simulink model "sampleModel1810_2"  (R2023a)
settings: Solver=VariableStepAuto  StartTime=0.0  StopTime=10.0  RelTol=1e-3
libraries: hdlsllib x6, simulink x4
settings Model: Creator=user1  LastModifiedBy=user1

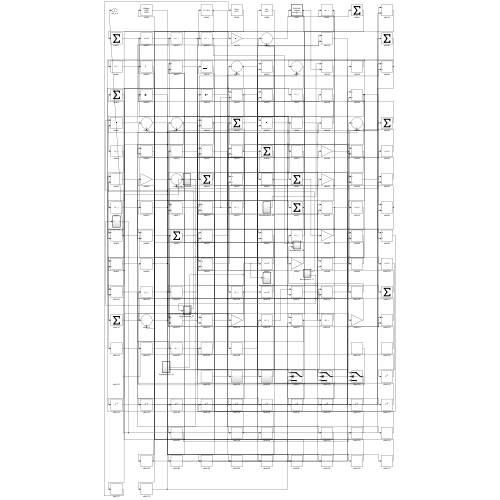
[thumbnail: Simulink's stored preview of the top-level diagram]
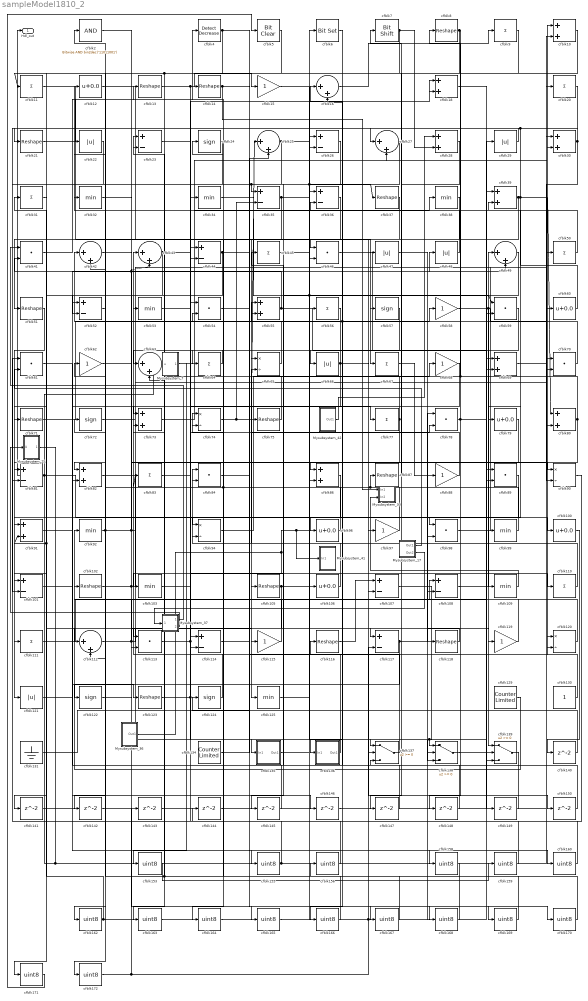
== system sampleModel1810_2 ==
  Mysubsystem_17 : Subsystem  TreatAsAtomicUnit=on  RTWFcnName=Mysubsystem_17
      settings: RTWFcnNameOpts=User specified  RTWFileNameOpts=Use function name
  Mysubsystem_25 : Subsystem  TreatAsAtomicUnit=on  RTWFcnName=Mysubsystem_25
      settings: RTWFcnNameOpts=User specified  RTWFileNameOpts=Use function name
  Mysubsystem_30 : Subsystem  TreatAsAtomicUnit=on  RTWFcnName=Mysubsystem_30
      settings: RTWFcnNameOpts=User specified  RTWFileNameOpts=Use function name
  Mysubsystem_36 : Subsystem  TreatAsAtomicUnit=on  RTWFcnName=Mysubsystem_36
      settings: RTWFcnNameOpts=User specified  RTWFileNameOpts=Use function name
  Mysubsystem_37 : Subsystem  TreatAsAtomicUnit=on  RTWFcnName=Mysubsystem_37
      settings: RTWFcnNameOpts=User specified  RTWFileNameOpts=Use function name
  Mysubsystem_41 : Subsystem  TreatAsAtomicUnit=on  RTWFcnName=Mysubsystem_41
      settings: RTWFcnNameOpts=User specified  RTWFileNameOpts=Use function name
  Mysubsystem_42 : Subsystem  TreatAsAtomicUnit=on  RTWFcnName=Mysubsystem_42
      settings: RTWFcnNameOpts=User specified  RTWFileNameOpts=Use function name
  Mysubsystem_7 : Subsystem  TreatAsAtomicUnit=on  RTWFcnName=Mysubsystem_7
      settings: RTWFcnNameOpts=User specified  RTWFileNameOpts=Use function name
  cfblk{10,18,28,30,39,55,69,73,80,82,86,91} (12 alike) : Sum  OutDataTypeStr=uint8
  cfblk{12,60,79,96,100,106} (6 alike) : Bias  Bias=0.0  SaturateOnIntegerOverflow=off
  cfblk{23,26,35..36,44,52,81,101,107..108,114,117} (12 alike) : Sum  Inputs=+-  OutDataTypeStr=uint8
  cfblk{8,13..14,21,37,51,71,75,87,102,105,116,118,123} (14 alike) : Reshape
  cfblk{32,34,38,53,92,99,103,109,125} (9 alike) : MinMax  OutDataTypeStr=uint8
  cfblk{9,11,20,31,45,50,56,64,67,77,83,110..111} (13 alike) : Sum  Inputs=+  OutDataTypeStr=uint8
  cfblk{16,25,27,42..43,49,63,112} (8 alike) : Sum  Inputs=|++  OutDataTypeStr=uint8
  cfblk{41,46,54,59,61,70,78,84,89,98,113} (11 alike) : DotProduct  OutDataTypeStr=uint8
  cfblk{15,58,62,68,88,97,115,119} (8 alike) : Gain  OutDataTypeStr=uint8
  cfblk{65,74,90,94,120} (5 alike) : Product  Inputs=*/  OutDataTypeStr=uint8  RndMeth=Zero  SaturateOnIntegerOverflow=on
  cfblk{22,29,47..48,66,121} (6 alike) : Abs  OutDataTypeStr=uint8  SaturateOnIntegerOverflow=off
  cfblk{24,57,72,122,124} (5 alike) : Signum
  cfblk129 : hdlsllib/Sources/Counter Limited  uplimit=7  tsamp=-1
  cfblk130 : Constant  OutDataTypeStr=uint8  SampleTime=-1
  cfblk131 : Ground
  cfblk134 : hdlsllib/Sources/Counter Limited  uplimit=7  tsamp=-1
  cfblk135 : Subsystem
      settings: LibrarySourceBlock=|
      | hdlsllib/Ports &
      | Subsystems/Subsystem
  cfblk136 : Subsystem
      settings: LibrarySourceBlock=|
      | hdlsllib/Ports &
      | Subsystems/Subsystem
  cfblk137 : Switch  OutDataTypeStr=uint8  SaturateOnIntegerOverflow=off  InputSameDT=off
  cfblk138 : Switch  OutDataTypeStr=uint8  SaturateOnIntegerOverflow=off  InputSameDT=off
  cfblk139 : Switch  OutDataTypeStr=uint8  SaturateOnIntegerOverflow=off  InputSameDT=off
  cfblk{140..150} (11 alike) : Delay  SampleTime=1
  cfblk{153,155..156,158..160,162..172} (17 alike) : DataTypeConversion  OutDataTypeStr=uint8  SaturateOnIntegerOverflow=off  RndMeth=Floor
  cfblk2 : simulink/Logic and Bit Operations/Bitwise Operator  logicop=AND  UseBitMask=on  BitMask=bin2dec('11011001')  BitMaskRealWorld=Stored Integer
      settings: LibrarySourceBlock=|
      | hdlsllib/Logic and Bit
      | Operations/Bitwise
      | Operator
  cfblk4 : simulink/Logic and Bit Operations/Detect Decrease  vinit=0.0  OutDataTypeStr=uint8
      settings: LibrarySourceBlock=|
      | hdlsllib/Logic and Bit
      | Operations/Detect
      | Decrease
  cfblk5 : simulink/Logic and Bit Operations/Bit Clear  iBit=0
      settings: LibrarySourceBlock=|
      | hdlsllib/Logic and Bit
      | Operations/Bit Clear
  cfblk6 : simulink/Logic and Bit Operations/Bit Set  iBit=0
      settings: LibrarySourceBlock=|
      | hdlsllib/Logic and Bit
      | Operations/Bit Set
  cfblk7 : hdlsllib/Logic and Bit Operations/Bit Shift  mode=Shift Left Logical  N=0
  Hdl_out : Outport  OutDataTypeStr=uint8
  wires:
  cfblk116/1 -> cfblk107/1
  cfblk82/1 -> cfblk135/1(In1)
  cfblk9/1 -> cfblk11/1, cfblk73/1
  cfblk65/1 -> cfblk42/1
  cfblk130/1 -> cfblk10/1
  cfblk67/1 -> cfblk88/1
  cfblk39/1 -> cfblk80/1, cfblk99/1, cfblk94/1
  cfblk11/1 -> cfblk67/1
  cfblk59/1 -> cfblk125/1
  cfblk124/1 -> cfblk43/1
  cfblk73/1 -> cfblk38/1
  cfblk36/1 -> cfblk46/1
  cfblk51/1 -> cfblk121/1
  cfblk108/1 -> cfblk49/1
  cfblk86/1 -> cfblk111/1
  cfblk74/1 -> cfblk25/1, cfblk35/2
  cfblk92/1 -> cfblk43/2, cfblk49/2, cfblk137/1, cfblk72/1
  cfblk57/1 -> cfblk66/1
  cfblk48/1 -> cfblk12/1
  cfblk58/1 -> cfblk139/1, cfblk60/1
  cfblk4/1 -> cfblk91/1, cfblk170/1
  cfblk129/1 -> cfblk92/1
  cfblk134/1 -> cfblk116/1
  cfblk99/1 -> cfblk87/1, cfblk83/1
  cfblk97/1 -> cfblk42/2
  cfblk70/1 -> cfblk16/1, cfblk23/1
  cfblk106/1 -> cfblk84/1
  cfblk38/1 -> cfblk65/1
  cfblk98/1 -> cfblk30/1
  cfblk16/1 -> cfblk9/1
  cfblk80/1 -> cfblk45/1, cfblk8/1, cfblk136/1(In1)
  cfblk7/1 -> cfblk82/1, cfblk28/2
  cfblk91/1 -> cfblk48/1
  cfblk81/1 -> cfblk100/1, Hdl_out/1
  cfblk30/1 -> cfblk27/1, cfblk90/2
  cfblk83/1 -> cfblk18/1
  cfblk138/1 -> cfblk120/1
  cfblk5/1 -> cfblk172/1
  cfblk131/1 -> cfblk25/2
  cfblk29/1 -> cfblk21/1
  cfblk88/1 -> cfblk55/1
  cfblk21/1 -> cfblk4/1
  cfblk46/1 -> cfblk69/2
  cfblk24/1 -> cfblk81/1
  cfblk110/1 -> cfblk65/2
  cfblk111/1 -> cfblk29/1
  cfblk94/1 -> cfblk26/1
  cfblk69/1 -> cfblk70/1
  cfblk112/1 -> cfblk115/1, cfblk108/1
  cfblk34/1 -> cfblk97/1
  cfblk102/1 -> cfblk10/2, cfblk114/2
  cfblk63/1 -> cfblk27/2
  cfblk15/1 -> cfblk37/1, cfblk59/2
  cfblk89/1 -> cfblk162/1
  cfblk137/1 -> cfblk53/1
  cfblk12/1 -> cfblk107/2
  cfblk135/1(Out1) -> cfblk18/2
  cfblk52/1 -> cfblk112/1
  cfblk71/1 -> cfblk26/2
  cfblk25/1 -> cfblk81/2, cfblk47/1
  cfblk103/1 -> cfblk34/1
  cfblk53/1 -> cfblk114/1
  cfblk107/1 -> cfblk139/2
  cfblk55/1 -> cfblk118/1, cfblk41/2
  cfblk37/1 -> cfblk103/1
  cfblk32/1 -> cfblk169/1
  cfblk20/1 -> cfblk79/1, cfblk101/2
  cfblk31/1 -> cfblk101/1
  cfblk139/1 -> cfblk137/3
  cfblk44/1 -> cfblk71/1, cfblk160/1
  cfblk8/1 -> cfblk117/1, cfblk148/1
  cfblk117/1 -> cfblk78/1, cfblk122/1
  cfblk75/1 -> cfblk24/1
  cfblk64/1 -> cfblk63/1
  cfblk87/1 -> cfblk7/1
  cfblk123/1 -> cfblk138/1, cfblk139/3, cfblk78/2
  cfblk41/1 -> cfblk13/1
  cfblk105/1 -> cfblk68/1, cfblk141/1
  cfblk79/1 -> cfblk86/1
  cfblk125/1 -> cfblk56/1
  cfblk78/1 -> cfblk110/1, cfblk98/1
  cfblk47/1 -> cfblk119/1
  cfblk60/1 -> cfblk36/2
  cfblk118/1 -> cfblk113/1
  cfblk13/1 -> cfblk15/1, cfblk77/1
  cfblk120/1 -> cfblk75/1
  cfblk96/1 -> cfblk63/2, cfblk74/2
  cfblk114/1 -> cfblk120/2
  cfblk62/1 -> cfblk86/2
  cfblk66/1 -> cfblk82/2, cfblk64/1, cfblk150/1
  cfblk61/1 -> cfblk155/1
  cfblk23/1 -> cfblk96/1
  cfblk136/1(Out1) -> cfblk74/1
  cfblk50/1 -> cfblk39/2
  cfblk27/1 -> cfblk35/1, cfblk112/2
  cfblk113/1 -> cfblk44/2, cfblk138/3
  cfblk77/1 -> cfblk113/2, cfblk23/2
  cfblk14/1 -> Mysubsystem_30/1(In1), cfblk90/1
  cfblk45/1 -> cfblk109/1, cfblk59/1
  cfblk119/1 -> cfblk62/1
  cfblk101/1 -> cfblk123/1
  cfblk72/1 -> cfblk20/1
  cfblk115/1 -> cfblk14/1
  cfblk28/1 -> cfblk57/1
  cfblk26/1 -> cfblk105/1
  cfblk84/1 -> cfblk58/1
  cfblk43/1 -> cfblk52/2, cfblk108/2
  cfblk35/1 -> cfblk51/1, cfblk138/2
  cfblk100/1 -> cfblk140/1
  cfblk140/1 -> cfblk84/2
  cfblk141/1 -> cfblk70/2
  cfblk68/1 -> cfblk142/1
  cfblk142/1 -> cfblk46/2
  cfblk143/1 -> cfblk69/1
  cfblk90/1 -> cfblk144/1
  cfblk144/1 -> cfblk39/1
  cfblk49/1 -> cfblk145/1
  cfblk145/1 -> cfblk52/1
  cfblk121/1 -> cfblk146/1
  cfblk146/1 -> cfblk80/2
  cfblk10/1 -> cfblk147/1
  cfblk147/1 -> cfblk55/2
  cfblk148/1 -> cfblk16/2
  cfblk18/1 -> cfblk149/1
  cfblk149/1 -> cfblk36/1
  cfblk150/1 -> cfblk44/1
  cfblk155/1 -> cfblk94/2, cfblk50/1
  cfblk156/1 -> cfblk61/1
  cfblk54/1 -> cfblk158/1
  cfblk158/1 -> cfblk156/1
  cfblk153/1 -> cfblk159/1
  cfblk159/1 -> cfblk54/1
  cfblk160/1 -> cfblk54/2
  cfblk162/1 -> cfblk98/2, cfblk137/2, cfblk91/2, cfblk31/1
  cfblk163/1 -> cfblk89/1
  cfblk56/1 -> cfblk164/1
  cfblk164/1 -> cfblk89/2
  cfblk42/1 -> cfblk165/1
  cfblk165/1 -> cfblk6/1
  cfblk6/1 -> cfblk166/1
  cfblk166/1 -> cfblk124/1
  cfblk122/1 -> cfblk167/1
  cfblk167/1 -> cfblk2/1
  cfblk2/1 -> cfblk168/1
  cfblk168/1 -> cfblk102/1
  cfblk169/1 -> cfblk73/2, cfblk22/1
  cfblk170/1 -> cfblk32/1
  cfblk22/1 -> cfblk171/1
  cfblk171/1 -> cfblk5/1
  cfblk172/1 -> cfblk143/1, cfblk117/2
  Mysubsystem_7/1(Out1) -> cfblk153/1
  Mysubsystem_17/1(Out1) -> cfblk61/2
  Mysubsystem_25/1(Out1) -> Mysubsystem_7/1(u), cfblk106/1
  cfblk109/1 -> Mysubsystem_30/2(In2)
  Mysubsystem_36/1(Out1) -> Mysubsystem_41/1(In1), cfblk30/2, cfblk163/1
  Mysubsystem_17/2(Out2) -> Mysubsystem_37/1(In1)
  Mysubsystem_37/1(Out1) -> cfblk41/1
  Mysubsystem_37/2(Out2) -> Mysubsystem_25/1(U)
  Mysubsystem_42/1(Out1) -> cfblk28/1

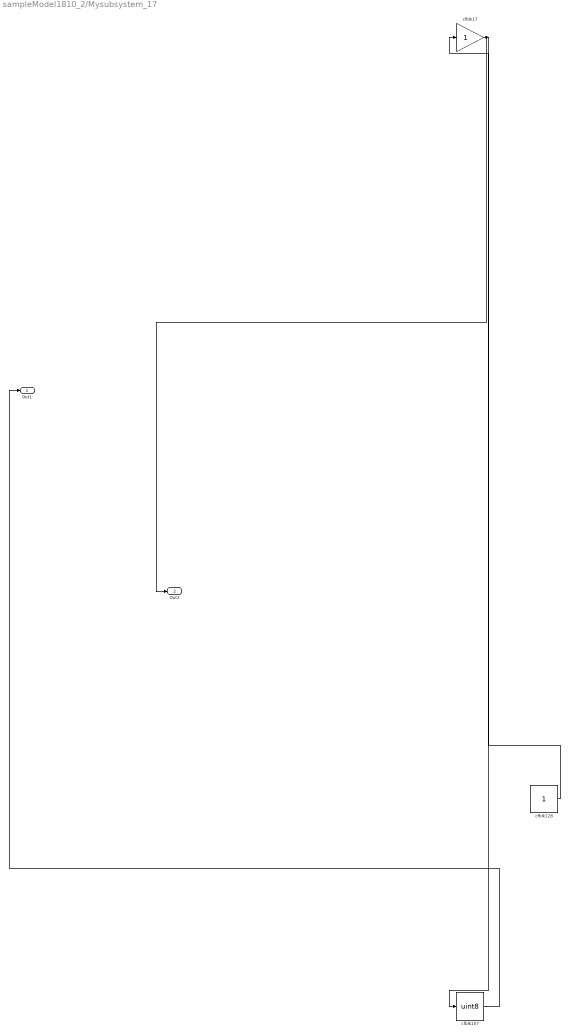
== system sampleModel1810_2/Mysubsystem_17 ==
  cfblk128 : Constant  SampleTime=-1
  cfblk157 : DataTypeConversion  OutDataTypeStr=uint8  SaturateOnIntegerOverflow=off  RndMeth=Floor
  cfblk17 : Gain
  Out1 : Outport
  Out2 : Outport  Port=2
  wires:
  cfblk17/1 -> Out2/1, cfblk157/1
  cfblk128/1 -> cfblk17/1
  cfblk157/1 -> Out1/1

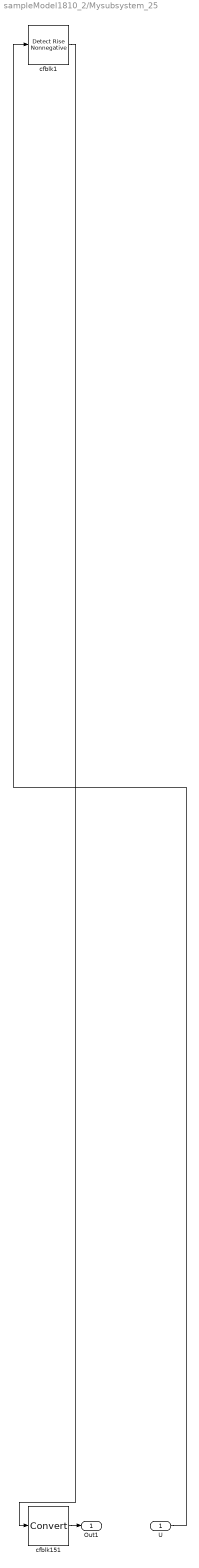
== system sampleModel1810_2/Mysubsystem_25 ==
  U : Inport
  cfblk1 : hdlsllib/Logic and Bit Operations/Detect Rise Nonnegative  vinit=0  OutDataTypeStr=boolean
  cfblk151 : DataTypeConversion  SaturateOnIntegerOverflow=off  RndMeth=Floor
  Out1 : Outport
  wires:
  cfblk1/1 -> cfblk151/1
  U/1 -> cfblk1/1
  cfblk151/1 -> Out1/1

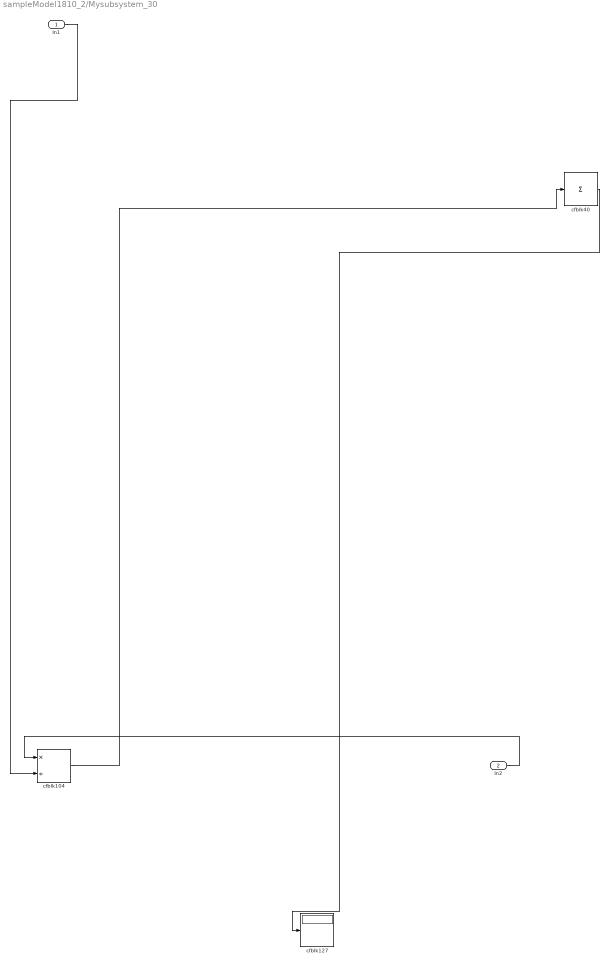
== system sampleModel1810_2/Mysubsystem_30 ==
  In1 : Inport
  In2 : Inport  Port=2
  cfblk104 : Product  Inputs=*/  RndMeth=Zero  SaturateOnIntegerOverflow=on
  cfblk127 : Display
  cfblk40 : Sum  Inputs=+
  wires:
  cfblk104/1 -> cfblk40/1
  cfblk40/1 -> cfblk127/1
  In1/1 -> cfblk104/2
  In2/1 -> cfblk104/1

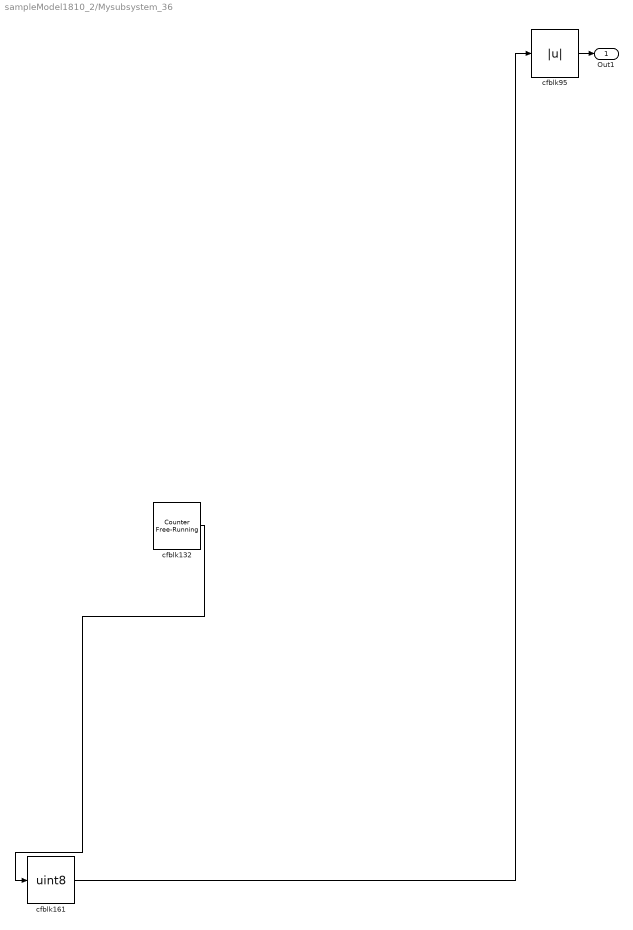
== system sampleModel1810_2/Mysubsystem_36 ==
  cfblk132 : hdlsllib/Sources/Counter Free-Running  NumBits=16  tsamp=-1
  cfblk161 : DataTypeConversion  OutDataTypeStr=uint8  SaturateOnIntegerOverflow=off  RndMeth=Floor
  cfblk95 : Abs  SaturateOnIntegerOverflow=off
  Out1 : Outport
  wires:
  cfblk161/1 -> cfblk95/1
  cfblk132/1 -> cfblk161/1
  cfblk95/1 -> Out1/1

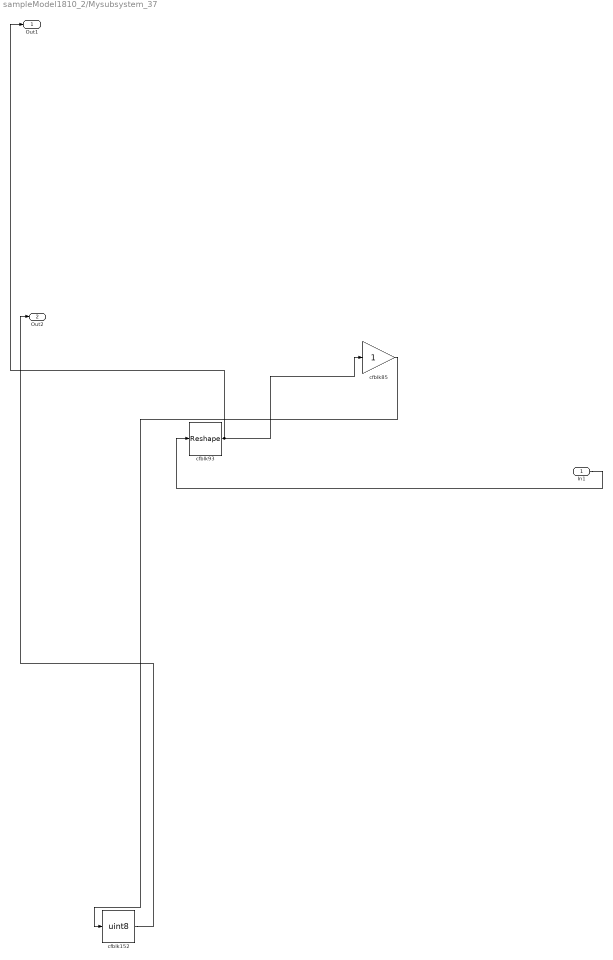
== system sampleModel1810_2/Mysubsystem_37 ==
  In1 : Inport
  cfblk152 : DataTypeConversion  OutDataTypeStr=uint8  SaturateOnIntegerOverflow=off  RndMeth=Floor
  cfblk85 : Gain
  cfblk93 : Reshape
  Out1 : Outport
  Out2 : Outport  Port=2
  wires:
  cfblk152/1 -> Out2/1
  cfblk85/1 -> cfblk152/1
  cfblk93/1 -> Out1/1, cfblk85/1
  In1/1 -> cfblk93/1

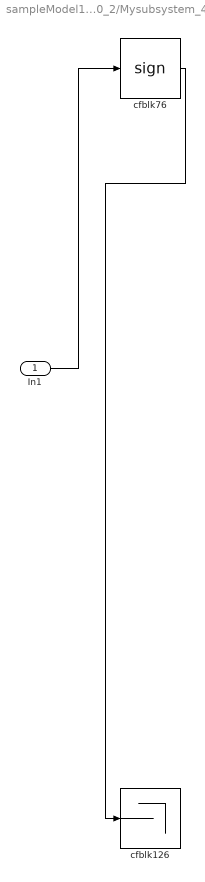
== system sampleModel1810_2/Mysubsystem_41 ==
  In1 : Inport
  cfblk126 : Terminator
  cfblk76 : Signum
  wires:
  cfblk76/1 -> cfblk126/1
  In1/1 -> cfblk76/1

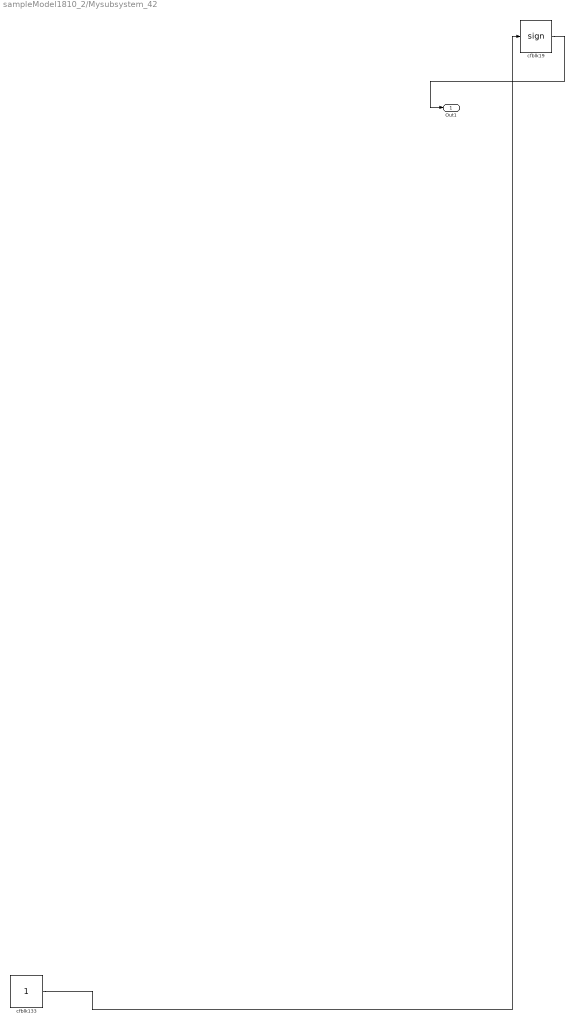
== system sampleModel1810_2/Mysubsystem_42 ==
  cfblk133 : Constant  SampleTime=-1
  cfblk19 : Signum
  Out1 : Outport
  wires:
  cfblk133/1 -> cfblk19/1
  cfblk19/1 -> Out1/1

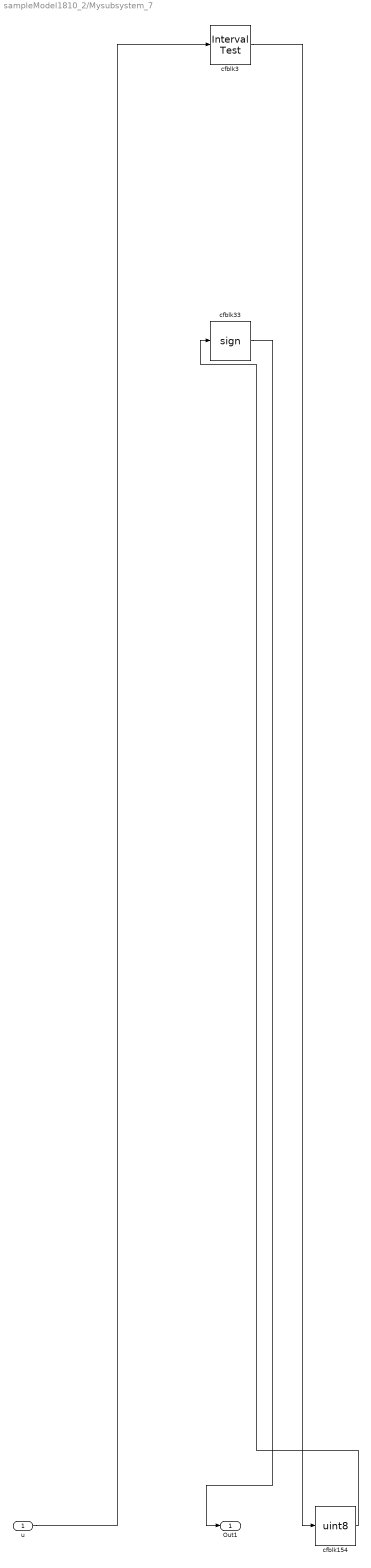
== system sampleModel1810_2/Mysubsystem_7 ==
  u : Inport
  cfblk154 : DataTypeConversion  OutDataTypeStr=uint8  SaturateOnIntegerOverflow=off  RndMeth=Floor
  cfblk3 : hdlsllib/Logic and Bit Operations/Interval Test  IntervalClosedRight=on  uplimit=0.5  IntervalClosedLeft=on  lowlimit=-0.5  OutDataTypeStr=boolean
  cfblk33 : Signum
  Out1 : Outport
  wires:
  u/1 -> cfblk3/1
  cfblk154/1 -> cfblk33/1
  cfblk3/1 -> cfblk154/1
  cfblk33/1 -> Out1/1

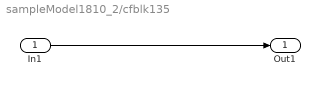
== system sampleModel1810_2/cfblk135 ==
  In1 : Inport
  Out1 : Outport
  wires:
  In1/1 -> Out1/1

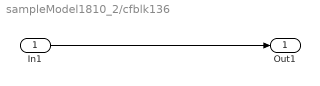
== system sampleModel1810_2/cfblk136 ==
  In1 : Inport
  Out1 : Outport
  wires:
  In1/1 -> Out1/1
